simulink model "CONTROLLER"  (R2023a)
settings: Solver=FixedStepAuto  StartTime=0.0  StopTime=10.0  FixedStep=0.01  RelTol=1e-3
libraries: simulink_extras x8
settings Model: Creator=james  LastModifiedBy=LENOVO
settings OptimizationCC: DefaultParameterBehavior=Inlined  UseDivisionForNetSlopeComputation=on  GainParamInheritBuiltInType=on  UseFloatMulNetSlope=on  InlineInvariantSignals=on  PassReuseOutputArgsAs=Individual arguments  ZeroExternalMemoryAtStartup=off  ZeroInternalMemoryAtStartup=off  NoFixptDivByZeroProtection=on  EfficientFloat2IntCast=on  LifeSpan=1  OptimizeBlockOrder=speed  DifferentSizesBufferReuse=on  EfficientTunableParamExpr=on
settings DebuggingCC: ParameterTunabilityLossMsg=error
settings HardwareCC: ProdBitPerPointer=32  ProdBitPerSizeT=32  ProdBitPerPtrDiffT=32  ProdLargestAtomicInteger=Long  ProdLargestAtomicFloat=Double  ProdWordSize=32  ProdLongLongMode=on  ProdHWDeviceType=ARM Compatible->ARM Cortex-M
settings SFSimCC: MATLABDynamicMemAlloc=off
settings RTWCC: Description=Embedded Coder  SystemTargetFile=ert.tlc  GenCodeOnly=on  TemplateMakefile=ert_default_tmf  GenerateReport=on  LaunchReport=on  DataTypeReplacement=CDataTypesFixedWidth
settings CodeAppCC: ForceParamTrailComments=on  IgnoreCustomStorageClasses=off  OperatorAnnotations=on  SimulinkDataObjDesc=on  SFDataObjDesc=on  CustomSymbolStrGlobalVar=rt$N$M  CustomSymbolStrType=$N$M  CustomSymbolStrFcn=$N$M$F  CustomSymbolStrMacro=$N$M  InsertBlockDesc=on
settings ERTTargetCC: TargetLangStandard=C99 (ISO)  GenerateSampleERTMain=on  IncludeMdlTerminateFcn=off  CombineSignalStateStructs=on  SupportAbsoluteTime=off  SupportComplex=off  SupportNonInlinedSFcns=on  InlinedParameterPlacement=NonHierarchical  ERTCustomFileTemplate=example_file_process.tlc  ERTFilePackagingFormat=CompactWithDataFile

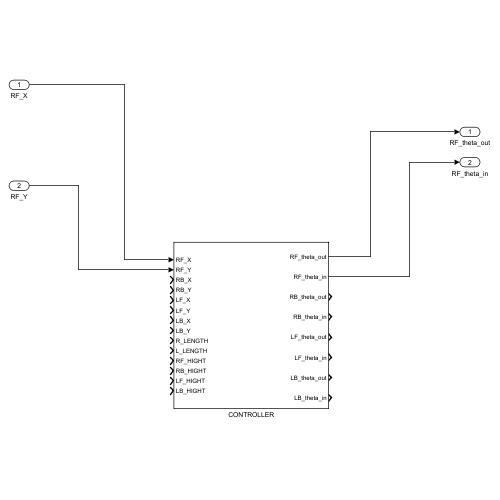
[thumbnail: Simulink's stored preview of the top-level diagram]
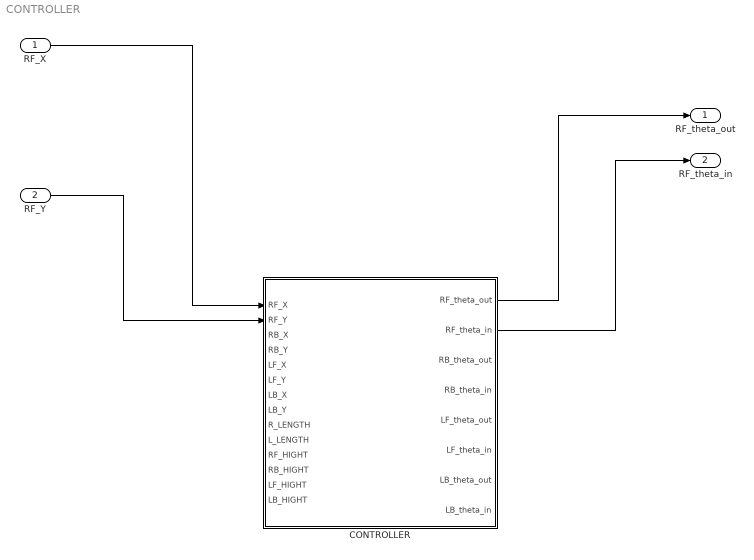
== system CONTROLLER ==
  RF_X : Inport  OutDataTypeStr=single
  RF_Y : Inport  Port=2  OutDataTypeStr=single
  CONTROLLER : Subsystem
  RF_theta_out : Outport  OutDataTypeStr=single
  RF_theta_in : Outport  Port=2  OutDataTypeStr=single
  wires:
  RF_X/1 -> CONTROLLER/1(RF_X)
  RF_Y/1 -> CONTROLLER/2(RF_Y)
  CONTROLLER/1(RF_theta_out) -> RF_theta_out/1
  CONTROLLER/2(RF_theta_in) -> RF_theta_in/1

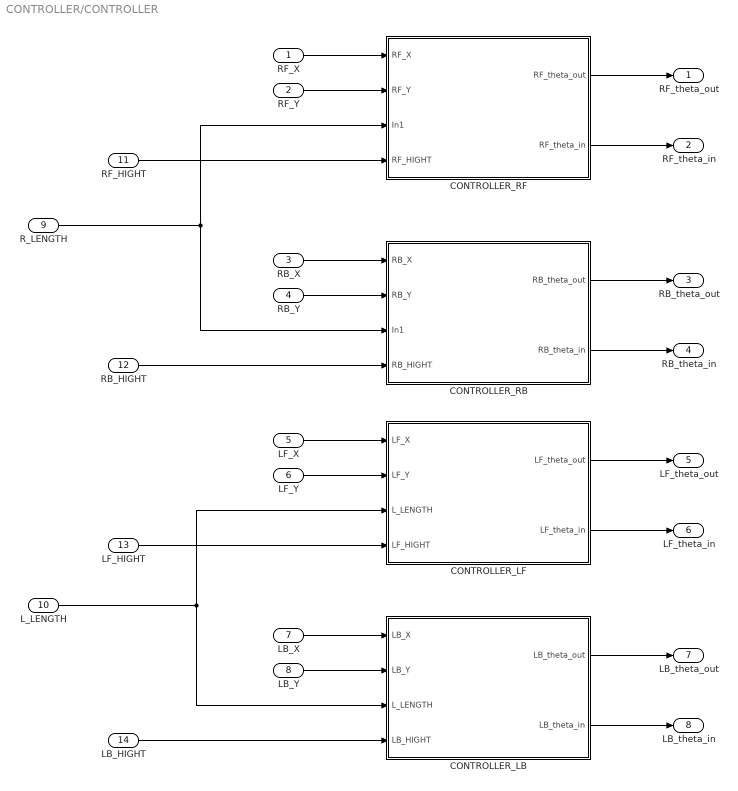
== system CONTROLLER/CONTROLLER ==
  RF_X : Inport  OutDataTypeStr=single
  RF_Y : Inport  Port=2  OutDataTypeStr=single
  RB_X : Inport  Port=3  OutDataTypeStr=single
  RB_Y : Inport  Port=4  OutDataTypeStr=single
  LF_X : Inport  Port=5  OutDataTypeStr=single
  LF_Y : Inport  Port=6  OutDataTypeStr=single
  LB_X : Inport  Port=7  OutDataTypeStr=single
  LB_Y : Inport  Port=8  OutDataTypeStr=single
  R_LENGTH : Inport  Port=9  OutDataTypeStr=single
  L_LENGTH : Inport  Port=10  OutDataTypeStr=single
  RF_HIGHT : Inport  Port=11  OutDataTypeStr=single
  RB_HIGHT : Inport  Port=12  OutDataTypeStr=single
  LF_HIGHT : Inport  Port=13  OutDataTypeStr=single
  LB_HIGHT : Inport  Port=14  OutDataTypeStr=single
  CONTROLLER_LB : Subsystem
  CONTROLLER_LF : Subsystem
  CONTROLLER_RB : Subsystem
  CONTROLLER_RF : Subsystem
  RF_theta_out : Outport  OutDataTypeStr=single
  RF_theta_in : Outport  Port=2  OutDataTypeStr=single
  RB_theta_out : Outport  Port=3  OutDataTypeStr=single
  RB_theta_in : Outport  Port=4  OutDataTypeStr=single
  LF_theta_out : Outport  Port=5  OutDataTypeStr=single
  LF_theta_in : Outport  Port=6  OutDataTypeStr=single
  LB_theta_out : Outport  Port=7  OutDataTypeStr=single
  LB_theta_in : Outport  Port=8  OutDataTypeStr=single
  wires:
  CONTROLLER_RF/2(RF_theta_in) -> RF_theta_in/1
  LB_Y/1 -> CONTROLLER_LB/2(LB_Y)
  RF_X/1 -> CONTROLLER_RF/1(RF_X)
  LF_X/1 -> CONTROLLER_LF/1(LF_X)
  CONTROLLER_RF/1(RF_theta_out) -> RF_theta_out/1
  CONTROLLER_LB/2(LB_theta_in) -> LB_theta_in/1
  CONTROLLER_LB/1(LB_theta_out) -> LB_theta_out/1
  RF_Y/1 -> CONTROLLER_RF/2(RF_Y)
  RB_X/1 -> CONTROLLER_RB/1(RB_X)
  RB_Y/1 -> CONTROLLER_RB/2(RB_Y)
  CONTROLLER_RB/1(RB_theta_out) -> RB_theta_out/1
  LB_X/1 -> CONTROLLER_LB/1(LB_X)
  CONTROLLER_RB/2(RB_theta_in) -> RB_theta_in/1
  CONTROLLER_LF/1(LF_theta_out) -> LF_theta_out/1
  CONTROLLER_LF/2(LF_theta_in) -> LF_theta_in/1
  LF_Y/1 -> CONTROLLER_LF/2(LF_Y)
  R_LENGTH/1 -> CONTROLLER_RB/3(In1), CONTROLLER_RF/3(In1)
  L_LENGTH/1 -> CONTROLLER_LB/3(L_LENGTH), CONTROLLER_LF/3(L_LENGTH)
  RF_HIGHT/1 -> CONTROLLER_RF/4(RF_HIGHT)
  RB_HIGHT/1 -> CONTROLLER_RB/4(RB_HIGHT)
  LF_HIGHT/1 -> CONTROLLER_LF/4(LF_HIGHT)
  LB_HIGHT/1 -> CONTROLLER_LB/4(LB_HIGHT)

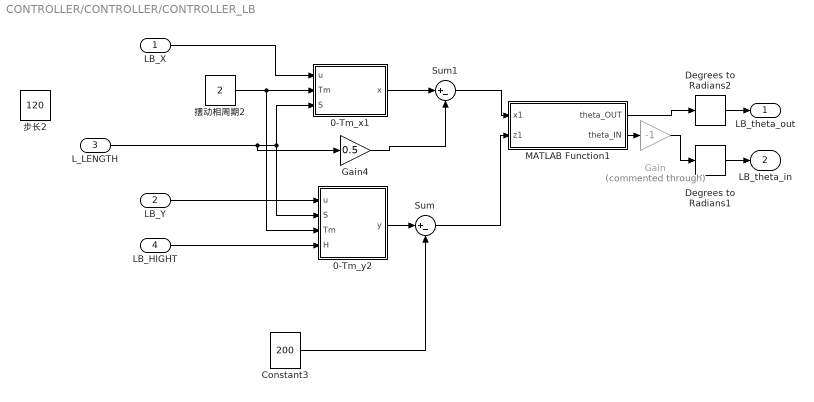
== system CONTROLLER/CONTROLLER/CONTROLLER_LB ==
  LB_X : Inport  OutDataTypeStr=single
  LB_Y : Inport  Port=2  OutDataTypeStr=single
  L_LENGTH : Inport  Port=3  OutDataTypeStr=single
  LB_HIGHT : Inport  Port=4  OutDataTypeStr=single
  0-Tm_x1 : MATLAB Function  TreatAsAtomicUnit=on
  0-Tm_y2 : MATLAB Function  TreatAsAtomicUnit=on
  Constant3 : Constant  Value=200
  Degrees to Radians1 : simulink_extras/Transformations/Degrees to Radians
  Degrees to Radians2 : simulink_extras/Transformations/Degrees to Radians
  Gain : Gain  Commented=through  Gain=-1
  Gain4 : Gain  Gain=0.5
  MATLAB Function1 : MATLAB Function  TreatAsAtomicUnit=on
  Sum : Sum  Inputs=|+-
  Sum1 : Sum  Inputs=|+-
  摆动相周期2 : Constant  Value=2
  步长2 : Constant  Value=120
  LB_theta_out : Outport  OutDataTypeStr=single
  LB_theta_in : Outport  Port=2  OutDataTypeStr=single
  wires:
  0-Tm_y2/1(y) -> Sum/1
  Gain4/1 -> Sum1/2
  MATLAB Function1/2(theta_IN) -> Gain/1
  摆动相周期2/1 -> 0-Tm_y2/3(Tm), 0-Tm_x1/2(Tm)
  L_LENGTH/1 -> Gain4/1, 0-Tm_y2/2(S), 0-Tm_x1/3(S)
  Gain/1 -> Degrees to Radians1/1
  LB_HIGHT/1 -> 0-Tm_y2/4(H)
  Sum/1 -> MATLAB Function1/2(z1)
  0-Tm_x1/1(x) -> Sum1/1
  Sum1/1 -> MATLAB Function1/1(x1)
  MATLAB Function1/1(theta_OUT) -> Degrees to Radians2/1
  LB_Y/1 -> 0-Tm_y2/1(u)
  LB_X/1 -> 0-Tm_x1/1(u)
  Constant3/1 -> Sum/2
  Degrees to Radians2/1 -> LB_theta_out/1
  Degrees to Radians1/1 -> LB_theta_in/1

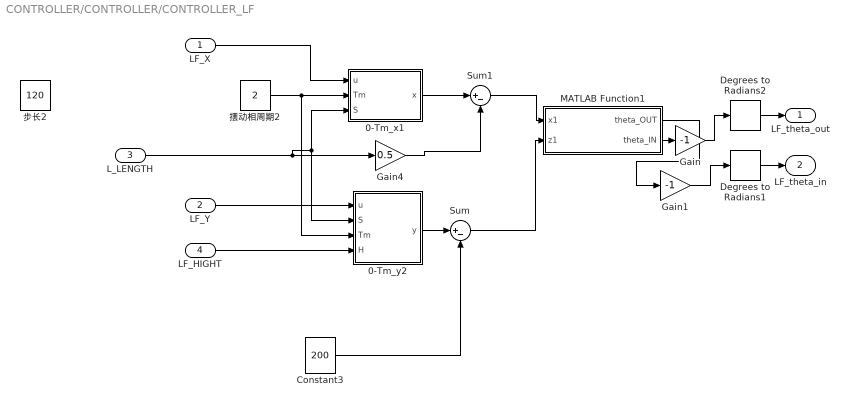
== system CONTROLLER/CONTROLLER/CONTROLLER_LF ==
  LF_X : Inport  OutDataTypeStr=single
  LF_Y : Inport  Port=2  OutDataTypeStr=single
  L_LENGTH : Inport  Port=3  OutDataTypeStr=single
  LF_HIGHT : Inport  Port=4  OutDataTypeStr=single
  0-Tm_x1 : MATLAB Function  TreatAsAtomicUnit=on
  0-Tm_y2 : MATLAB Function  TreatAsAtomicUnit=on
  Constant3 : Constant  Value=200
  Degrees to Radians1 : simulink_extras/Transformations/Degrees to Radians
  Degrees to Radians2 : simulink_extras/Transformations/Degrees to Radians
  Gain : Gain  Gain=-1
  Gain1 : Gain  Gain=-1
  Gain4 : Gain  Gain=0.5
  MATLAB Function1 : MATLAB Function  TreatAsAtomicUnit=on
  Sum : Sum  Inputs=|+-
  Sum1 : Sum  Inputs=|+-
  摆动相周期2 : Constant  Value=2
  步长2 : Constant  Value=120
  LF_theta_out : Outport  OutDataTypeStr=single
  LF_theta_in : Outport  Port=2  OutDataTypeStr=single
  wires:
  0-Tm_y2/1(y) -> Sum/1
  Gain4/1 -> Sum1/2
  MATLAB Function1/2(theta_IN) -> Gain/1
  摆动相周期2/1 -> 0-Tm_y2/3(Tm), 0-Tm_x1/2(Tm)
  L_LENGTH/1 -> 0-Tm_y2/2(S), 0-Tm_x1/3(S), Gain4/1
  Gain/1 -> Degrees to Radians2/1
  LF_HIGHT/1 -> 0-Tm_y2/4(H)
  Sum/1 -> MATLAB Function1/2(z1)
  0-Tm_x1/1(x) -> Sum1/1
  Sum1/1 -> MATLAB Function1/1(x1)
  MATLAB Function1/1(theta_OUT) -> Gain1/1
  LF_Y/1 -> 0-Tm_y2/1(u)
  LF_X/1 -> 0-Tm_x1/1(u)
  Constant3/1 -> Sum/2
  Degrees to Radians2/1 -> LF_theta_out/1
  Degrees to Radians1/1 -> LF_theta_in/1
  Gain1/1 -> Degrees to Radians1/1

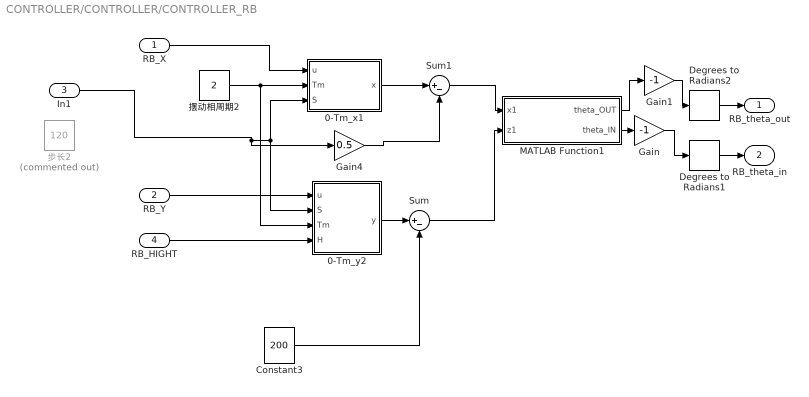
== system CONTROLLER/CONTROLLER/CONTROLLER_RB ==
  RB_X : Inport  OutDataTypeStr=single
  RB_Y : Inport  Port=2  OutDataTypeStr=single
  In1 : Inport  Port=3  OutDataTypeStr=single
  RB_HIGHT : Inport  Port=4  OutDataTypeStr=single
  0-Tm_x1 : MATLAB Function  TreatAsAtomicUnit=on
  0-Tm_y2 : MATLAB Function  TreatAsAtomicUnit=on
  Constant3 : Constant  Value=200
  Degrees to Radians1 : simulink_extras/Transformations/Degrees to Radians
  Degrees to Radians2 : simulink_extras/Transformations/Degrees to Radians
  Gain : Gain  Gain=-1
  Gain1 : Gain  Gain=-1
  Gain4 : Gain  Gain=0.5
  MATLAB Function1 : MATLAB Function  TreatAsAtomicUnit=on
  Sum : Sum  Inputs=|+-
  Sum1 : Sum  Inputs=|+-
  摆动相周期2 : Constant  Value=2
  步长2 : Constant  Commented=on  Value=120
  RB_theta_out : Outport  OutDataTypeStr=single
  RB_theta_in : Outport  Port=2  OutDataTypeStr=single
  wires:
  0-Tm_y2/1(y) -> Sum/1
  Gain4/1 -> Sum1/2
  MATLAB Function1/2(theta_IN) -> Gain/1
  摆动相周期2/1 -> 0-Tm_y2/3(Tm), 0-Tm_x1/2(Tm)
  In1/1 -> Gain4/1, 0-Tm_y2/2(S), 0-Tm_x1/3(S)
  Gain/1 -> Degrees to Radians1/1
  RB_HIGHT/1 -> 0-Tm_y2/4(H)
  Sum/1 -> MATLAB Function1/2(z1)
  0-Tm_x1/1(x) -> Sum1/1
  Sum1/1 -> MATLAB Function1/1(x1)
  MATLAB Function1/1(theta_OUT) -> Gain1/1
  RB_Y/1 -> 0-Tm_y2/1(u)
  RB_X/1 -> 0-Tm_x1/1(u)
  Constant3/1 -> Sum/2
  Degrees to Radians2/1 -> RB_theta_out/1
  Degrees to Radians1/1 -> RB_theta_in/1
  Gain1/1 -> Degrees to Radians2/1

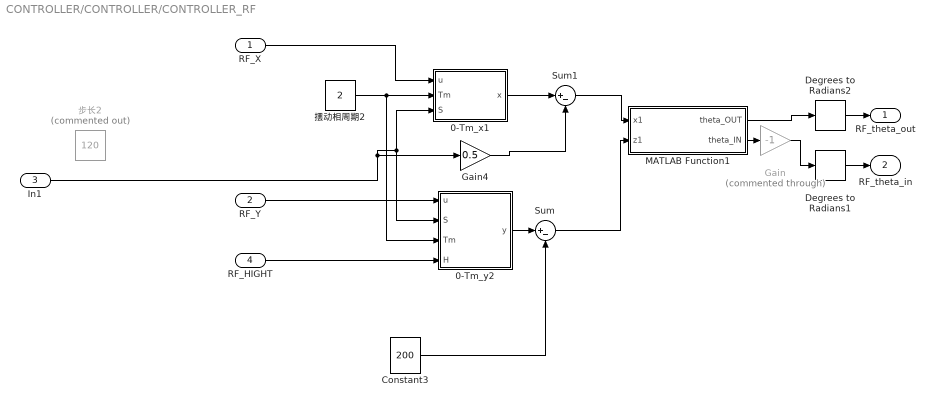
== system CONTROLLER/CONTROLLER/CONTROLLER_RF ==
  RF_X : Inport  OutDataTypeStr=single
  RF_Y : Inport  Port=2  OutDataTypeStr=single
  In1 : Inport  Port=3  OutDataTypeStr=single
  RF_HIGHT : Inport  Port=4  OutDataTypeStr=single
  0-Tm_x1 : MATLAB Function  TreatAsAtomicUnit=on
  0-Tm_y2 : MATLAB Function  TreatAsAtomicUnit=on
  Constant3 : Constant  Value=200
  Degrees to Radians1 : simulink_extras/Transformations/Degrees to Radians
  Degrees to Radians2 : simulink_extras/Transformations/Degrees to Radians
  Gain : Gain  Commented=through  Gain=-1
  Gain4 : Gain  Gain=0.5
  MATLAB Function1 : MATLAB Function  TreatAsAtomicUnit=on
  Sum : Sum  Inputs=|+-
  Sum1 : Sum  Inputs=|+-
  摆动相周期2 : Constant  Value=2
  步长2 : Constant  Commented=on  Value=120
  RF_theta_out : Outport  OutDataTypeStr=single
  RF_theta_in : Outport  Port=2  OutDataTypeStr=single
  wires:
  0-Tm_y2/1(y) -> Sum/1
  Gain4/1 -> Sum1/2
  MATLAB Function1/2(theta_IN) -> Gain/1
  摆动相周期2/1 -> 0-Tm_y2/3(Tm), 0-Tm_x1/2(Tm)
  In1/1 -> 0-Tm_y2/2(S), 0-Tm_x1/3(S), Gain4/1
  Gain/1 -> Degrees to Radians1/1
  RF_HIGHT/1 -> 0-Tm_y2/4(H)
  Sum/1 -> MATLAB Function1/2(z1)
  0-Tm_x1/1(x) -> Sum1/1
  Sum1/1 -> MATLAB Function1/1(x1)
  MATLAB Function1/1(theta_OUT) -> Degrees to Radians2/1
  RF_Y/1 -> 0-Tm_y2/1(u)
  RF_X/1 -> 0-Tm_x1/1(u)
  Constant3/1 -> Sum/2
  Degrees to Radians2/1 -> RF_theta_out/1
  Degrees to Radians1/1 -> RF_theta_in/1

== matlab function CONTROLLER/CONTROLLER_RF/0-Tm_x1 ==
  data: u input; x output; Tm input; S input
function x = fcn(u,Tm,S)

if u>0
    x =S*(u/Tm-1/(2*pi)*sin(2*pi*u/Tm));
else 
    u=-u;
     x =S*(u/Tm-1/(2*pi)*sin(2*pi*u/Tm));
end

== matlab function CONTROLLER/CONTROLLER_LB/0-Tm_y2 ==
  data: u input; y output; S input; Tm input; H input
function y = fcn(u,S,Tm,H)

n=4;
if u>0
    y=2*H*(u/Tm-1/(n*pi)*sin(n*pi*u/Tm)).*(u>=0&u<Tm/2)+2*H*(1-u/Tm+1/(n*pi)*sin(n*pi*u/Tm)).*(u>=Tm/2&u<Tm);;
else 
    y = single(0);
end

== matlab function CONTROLLER/CONTROLLER_LB/MATLAB Function1 ==
  data: x1 input; theta_OUT output; z1 input; theta_IN output
function [theta_OUT, theta_IN ] = fcn(x1, z1)

%#codegen


L1 = 100;
L2 = 180;

x = x1;
y = z1;

L = sqrt(x^2 + y^2);

theta_left =  rad2deg(asin(x/L));

theta_right = rad2deg( acos((L^2 + L1^2-L2^2)/(2*L1*L)));



theta_OUT = theta_right- theta_left ;

theta_IN = theta_right + theta_left;

== matlab function CONTROLLER/CONTROLLER_RF/0-Tm_y2 ==
  data: u input; y output; S input; Tm input; H input
function y = fcn(u,S,Tm,H)

n=4;
if u>0
    y=2*H*(u/Tm-1/(n*pi)*sin(n*pi*u/Tm)).*(u>=0&u<Tm/2)+2*H*(1-u/Tm+1/(n*pi)*sin(n*pi*u/Tm)).*(u>=Tm/2&u<Tm);;
else 
   
    y =single(0);
end

== matlab function CONTROLLER/CONTROLLER_RB/0-Tm_x1 ==
  data: u input; x output; Tm input; S input
function x = fcn(u,Tm,S)

if u>0
    x =S*(u/Tm-1/(2*pi)*sin(2*pi*u/Tm));
else 
    u=-u;
     x =S*(u/Tm-1/(2*pi)*sin(2*pi*u/Tm));
end

== matlab function CONTROLLER/CONTROLLER_RB/0-Tm_y2 ==
  data: u input; y output; S input; Tm input; H input
function y = fcn(u,S,Tm,H)

n=4;
if u>0
    y=2*H*(u/Tm-1/(n*pi)*sin(n*pi*u/Tm)).*(u>=0&u<Tm/2)+2*H*(1-u/Tm+1/(n*pi)*sin(n*pi*u/Tm)).*(u>=Tm/2&u<Tm);;
else 
    y = single(0);
end

== matlab function CONTROLLER/CONTROLLER_RB/MATLAB Function1 ==
  data: x1 input; theta_OUT output; z1 input; theta_IN output
function [theta_OUT, theta_IN ] = fcn(x1, z1)

%#codegen


L1 = 100;
L2 = 180;

x = x1;
y = z1;

L = sqrt(x^2 + y^2);

theta_left =  rad2deg(asin(x/L));

theta_right = rad2deg( acos((L^2 + L1^2-L2^2)/(2*L1*L)));



theta_OUT = theta_right- theta_left ;

theta_IN = theta_right + theta_left;

== matlab function CONTROLLER/CONTROLLER_RF/MATLAB Function1 ==
  data: x1 input; theta_OUT output; z1 input; theta_IN output
function [theta_OUT, theta_IN ] = fcn(x1, z1)

%#codegen


L1 = 100;
L2 = 180;

x = x1;
y = z1;

L = sqrt(x^2 + y^2);

theta_left =  rad2deg(asin(x/L));

theta_right = rad2deg( acos((L^2 + L1^2-L2^2)/(2*L1*L)));



theta_OUT = theta_right- theta_left ;

theta_IN = theta_right + theta_left;

== matlab function CONTROLLER/CONTROLLER_LF/0-Tm_x1 ==
  data: u input; x output; Tm input; S input
function x = fcn(u,Tm,S)

if u>0
    x =S*(u/Tm-1/(2*pi)*sin(2*pi*u/Tm));
else 
    u=-u;
     x =S*(u/Tm-1/(2*pi)*sin(2*pi*u/Tm));
end

== matlab function CONTROLLER/CONTROLLER_LF/0-Tm_y2 ==
  data: u input; y output; S input; Tm input; H input
function y = fcn(u,S,Tm,H)

n=4;
if u>0
    y=2*H*(u/Tm-1/(n*pi)*sin(n*pi*u/Tm)).*(u>=0&u<Tm/2)+2*H*(1-u/Tm+1/(n*pi)*sin(n*pi*u/Tm)).*(u>=Tm/2&u<Tm);;
else 
    y = single(0);
end

== matlab function CONTROLLER/CONTROLLER_LF/MATLAB Function1 ==
  data: x1 input; theta_OUT output; z1 input; theta_IN output
function [theta_OUT, theta_IN ] = fcn(x1, z1)

%#codegen


L1 = 100;
L2 = 180;

x = x1;
y = z1;

L = sqrt(x^2 + y^2);

theta_left =  rad2deg(asin(x/L));

theta_right = rad2deg( acos((L^2 + L1^2-L2^2)/(2*L1*L)));



theta_OUT = theta_right- theta_left ;

theta_IN = theta_right + theta_left;

== matlab function CONTROLLER/CONTROLLER_LB/0-Tm_x1 ==
  data: u input; x output; Tm input; S input
function x = fcn(u,Tm,S)

if u>0
    x =S*(u/Tm-1/(2*pi)*sin(2*pi*u/Tm));
else 
    u=-u;
     x =S*(u/Tm-1/(2*pi)*sin(2*pi*u/Tm));
end
